simulink model "SwingEqn"  (Simulink 7.3)
settings: Solver=ode4  StartTime=0.0  StopTime=100  FixedStep=0.001  RelTol=1e-3
libraries: powerlib_extras x1
settings Model: Creator=Apps  LastModifiedBy=Apps

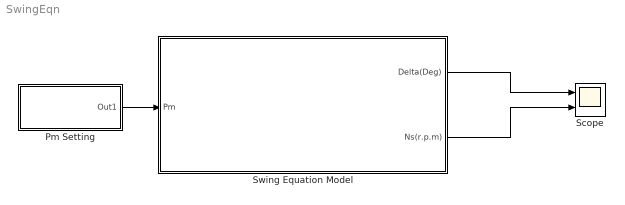
== system SwingEqn ==
  Pm Setting : Subsystem  mask{Pm1=100, Pm2=520}
      mask prompts: Pm1 "Initial Mechanical Input (MW)"; Pm2 "Final Mechanical Input (MW)"
  Scope : Scope  NumInputPorts=2
      settings: YMin=-5~-5  YMax=5~5  SampleTime=0.0001
  Swing Equation Model : Subsystem  mask{S=611.76, H=3.4, Pemax=813.65, Dd=0.008}
      mask prompts: S "Rating (MVA)"; H "Inertia Constant (MJ/MVA)"; Pemax "Max Power Capability (MW)"; Dd "Damping Torque co-eff (N-m-sec)"
  wires:
  Swing Equation Model/1(Delta(Deg)) -> Scope/1
  Swing Equation Model/2(Ns(r.p.m)) -> Scope/2
  Pm Setting/1(Out1) -> Swing Equation Model/1(Pm)

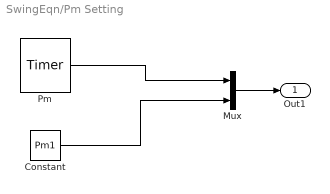
== system SwingEqn/Pm Setting ==
  Constant : Constant  Value=Pm1  OutDataType=fixdt(1, 16)  OutScaling=2^0
  Mux : Mux  Inputs=2
  Pm : powerlib_extras/Control  Blocks/Timer  DialogController=POWERSYS.PowerSysDialog  SystemSampleTime=-1  t=[ 0 5 ]  e=[ Pm1 Pm2 ]
  Out1 : Outport  OutDataType=fixdt(1, 16)  OutScaling=2^0
  wires:
  Mux/1 -> Out1/1
  Pm/1 -> Mux/1
  Constant/1 -> Mux/2

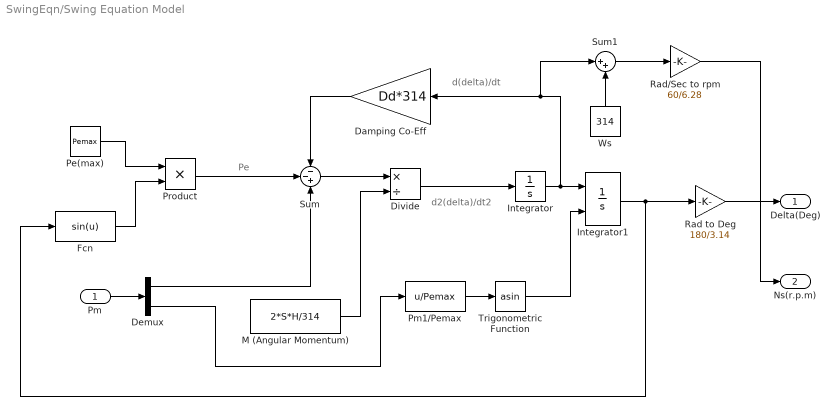
== system SwingEqn/Swing Equation Model ==
  note: Pe
  note: d(delta)/dt
  note: d2(delta)/dt2
  Pm : Inport  OutDataType=fixdt(1, 16)  OutScaling=2^0
  Damping Co-Eff : Gain  Gain=Dd*314  ParameterDataType=fixdt(1, 16)  ParameterScaling=2^0  OutDataType=fixdt(1, 16)  OutScaling=2^0
  Demux : Demux  Outputs=2
  Divide : Product  Inputs=*/  OutDataType=fixdt(1, 16)  OutScaling=2^-10
  Fcn : Fcn  Expr=sin(u)
  Integrator : Integrator
  Integrator1 : Integrator  InitialConditionSource=external  InitialCondition=0.1374
  M (Angular Momentum) : Constant  Value=2*S*H/314  OutDataType=fixdt(1, 16)  OutScaling=2^0
  Pe(max) : Constant  Value=Pemax  OutDataType=fixdt(1, 16)  OutScaling=2^0
  Pm1/Pemax : Fcn  Expr=u/Pemax
  Product : Product  OutDataType=fixdt(1, 16)  OutScaling=2^0  RndMeth=Zero
  Rad to Deg : Gain  Gain=180/3.14  ParameterDataType=fixdt(1, 16)  ParameterScaling=2^0  OutDataType=fixdt(1, 16)  OutScaling=2^0
  "Rad/Sec to rpm " : Gain  Gain=60/6.28  ParameterDataType=fixdt(1, 16)  ParameterScaling=2^0  OutDataType=fixdt(1, 16)  OutScaling=2^0
  Sum : Sum  Inputs=--+  OutDataType=fixdt(1, 16)  OutScaling=2^0
  Sum1 : Sum  Inputs=|++  OutDataType=fixdt(1, 16)  OutScaling=2^0
  Trigonometric Function : Trigonometry  Operator=asin
  Ws : Constant  Value=314  OutDataType=fixdt(1, 16)  OutScaling=2^0
  Delta(Deg) : Outport  OutDataType=fixdt(1, 16)  OutScaling=2^0
  Ns(r.p.m) : Outport  Port=2  OutDataType=fixdt(1, 16)  OutScaling=2^0
  wires:
  Pe(max)/1 -> Product/1
  Fcn/1 -> Product/2
  Sum/1 -> Divide/1
  M (Angular Momentum)/1 -> Divide/2
  Divide/1 -> Integrator/1
  Integrator/1 -> Integrator1/1, Damping Co-Eff/1, Sum1/1
  Integrator1/1 -> Fcn/1, Rad to Deg/1
  Product/1 -> Sum/2
  Damping Co-Eff/1 -> Sum/1
  Rad to Deg/1 -> Delta(Deg)/1
  Pm1/Pemax/1 -> Trigonometric Function/1
  Trigonometric Function/1 -> Integrator1/2
  Ws/1 -> Sum1/2
  Sum1/1 -> "Rad/Sec to rpm "/1
  "Rad/Sec to rpm "/1 -> Ns(r.p.m)/1
  Pm/1 -> Demux/1
  Demux/1 -> Sum/3
  Demux/2 -> Pm1/Pemax/1
